simulink model "eAgriBot_V4"  (R2022b)
settings: Solver=ode3  StartTime=0.0  StopTime=t_sim  FixedStep=step_size  RelTol=1e-3
values from neighbouring files (symbols this model uses):
  accel = 0.1*9.81    (= 0.981)    [Run_eAgriBot_V4.m]
  B_tines = 5    [Run_eAgriBot_V4.m]
  brake_bias = 1    [Run_eAgriBot_V4.m]
  c = 6100    [Run_eAgriBot_V4.m]
  decel = 0.15*9.81    (= 1.4715)    [Run_eAgriBot_V4.m]
  decel_begin_dist = total_dist_target    (= 100)    [Run_eAgriBot_V4.m]
  drivetype = 3    [Run_eAgriBot_V4.m]
  effmap = [0.5 0.586 0.723 0.778 0.614 0.604 0.6 0.584 0.709 0.658 0.586 0.688 ... (121 elements, 11x11)]    [EM_effmap_generic.mat]
  end_delay = 4    [Run_eAgriBot_V4.m]
  F_tines = 5    [Run_eAgriBot_V4.m]
  Fb_max = m*g    (= 5101.2)    [Run_eAgriBot_V4.m]
  FT_c_x_rel = l_f    (= 0.645)    [Run_eAgriBot_V4.m]
  FT_c_z_rel = R_u-h_CoG    (= -0.2825)    [Run_eAgriBot_V4.m]
  g = 9.81    [Run_eAgriBot_V4.m]
  gb_eff = 0.98    [Run_eAgriBot_V4.m]
  ground_coh = c*ones(length(ground_points),1)    [Run_eAgriBot_V4.m]
  ground_dens = gamma_s*ones(length(ground_points),1)    [Run_eAgriBot_V4.m]
  ground_height = zeros(length(ground_points),1)    [Run_eAgriBot_V4.m]
  ground_kxy = k_xy*ones(length(ground_points),1)    [Run_eAgriBot_V4.m]
  ground_res = 0.01    [Run_eAgriBot_V4.m]
  Har_back_tip_x_rel = Har_back_top_x_rel+Har_tine_length*cos(Har_angle)    [Run_eAgriBot_V4.m]
  Har_back_tip_z_rel = abs(Hook_z_rel)-h_CoG-Har_tine_depth    [Run_eAgriBot_V4.m]
  Har_back_top_x_rel = -2.0    (= -2)    [Run_eAgriBot_V4.m]
  Har_back_top_z_rel = Har_back_tip_z_rel+Har_tine_length*sin(Har_angle)    [Run_eAgriBot_V4.m]
  Har_front_tip_x_rel = Har_front_top_x_rel+Har_tine_length*cos(Har_angle)    [Run_eAgriBot_V4.m]
  Har_front_tip_z_rel = abs(Hook_z_rel)-h_CoG-Har_tine_depth    [Run_eAgriBot_V4.m]
  Har_front_top_x_rel = -1.2    [Run_eAgriBot_V4.m]
  Har_front_top_z_rel = Har_front_tip_z_rel+Har_tine_length*sin(Har_angle)    [Run_eAgriBot_V4.m]
  Har_tine_length = 0.25    [Run_eAgriBot_V4.m]
  Har_tine_width = 0.02    [Run_eAgriBot_V4.m]
  Har_tire_rad = 0.5842/2    (= 0.2921)    [Run_eAgriBot_V4.m]
  Har_tire_x_rel = -1.5    [Run_eAgriBot_V4.m]
  Har_tire_z_rel = abs(Hook_z_rel)-h_CoG+Har_tire_rad    [Run_eAgriBot_V4.m]
  Hook_x_rel = l_f-l-0.4    (= -1.045)    [Run_eAgriBot_V4.m]
  Hook_z_rel = -0.3    [Run_eAgriBot_V4.m]
  i_front = 17.9542    [Run_eAgriBot_V4.m]
  I_gain = 0.0    (= 0)    [Run_eAgriBot_V4.m]
  i_rear = 17.9542    [Run_eAgriBot_V4.m]
  I_y = 150    [Run_eAgriBot_V4.m]
  I_y_tool = 20    [Run_eAgriBot_V4.m]
  index_init = round(FT_init_exit_x/ground_res)+1    [Run_eAgriBot_V4.m]
  init_CoG_height = h_CoG-0.001    (= 0.599)    [Run_eAgriBot_V4.m]
  init_CoG_v_z = 0    [Run_eAgriBot_V4.m]
  init_omega = 0    [Run_eAgriBot_V4.m]
  init_theta = 0    [Run_eAgriBot_V4.m]
  J_front = J_drive    (= 15)    [Run_eAgriBot_V4.m]
  J_harrow = 1    [Run_eAgriBot_V4.m]
  J_rear = J_drive    (= 15)    [Run_eAgriBot_V4.m]
  k_d = 50e2    (= 5000)    [Run_eAgriBot_V4.m]
  k_d_har = 50e2    (= 5000)    [Run_eAgriBot_V4.m]
  m = 520    [Run_eAgriBot_V4.m]
  m_tool = 200    [Run_eAgriBot_V4.m]
  main_cycle_delay = 5    [Run_eAgriBot_V4.m]
  mu = 0.35    [Run_eAgriBot_V4.m]
  omega_tool_init = 0    [Run_eAgriBot_V4.m]
  P_aux = 200    [Run_eAgriBot_V4.m]
  P_gain = 1.0    (= 1)    [Run_eAgriBot_V4.m]
  pack_Ah = 360    [Battery_data_V5_Kokam_NMC.mat]
  pack_R_charge = [0.00267222222222 0.00267222222222 0.00317777777778 0.00310555555556 0.0026 0.00281666666667 0.00332222222222 0.00353888888889 0.00325 0.00382777777778 0.00382777777778]    [Battery_data_V5_Kokam_NMC.mat]
  pack_R_discharge = [0.00267222222222 0.00267222222222 0.00317777777778 0.00310555555556 0.0026 0.00281666666667 0.00332222222222 0.00353888888889 0.00325 0.00382777777778 0.00382777777778]    [Battery_data_V5_Kokam_NMC.mat]
  pack_VOC = [54.509 52.351 50.895 49.556 48.477 47.645 47.008 46.449 45.825 44.941 44.941]    [Battery_data_V5_Kokam_NMC.mat]
  params2 = [exit_angle reso theta_m_max s_d_tol po]    [Run_eAgriBot_V4.m]
  phi = 26.6    [Run_eAgriBot_V4.m]
  pre_accel = 0.1*9.81    (= 0.981)    [Run_eAgriBot_V4.m]
  pre_decel = 0.15*9.81    (= 1.4715)    [Run_eAgriBot_V4.m]
  pre_decel_begin_dist = pre_dist_target-pre_decel_dist    (= 2.34454218631)    [Run_eAgriBot_V4.m]
  pre_vel = 5    [Run_eAgriBot_V4.m]
  r_front = R_u    (= 0.3175)    [Run_eAgriBot_V4.m]
  r_rear = R_u    (= 0.3175)    [Run_eAgriBot_V4.m]
  rho_t = gamma_s/9.81    (= 1664.01630989)    [Run_eAgriBot_V4.m]
  RT_c_x_rel = l_f-l    (= -0.645)    [Run_eAgriBot_V4.m]
  RT_c_z_rel = R_u-h_CoG    (= -0.2825)    [Run_eAgriBot_V4.m]
  s_init = 3    [Run_eAgriBot_V4.m]
  simu_max_time = cycle_total_time*4    (= 259.930519878)    [Run_eAgriBot_V4.m]
  slip_init = 0    [Run_eAgriBot_V4.m]
  slip_ub = r_rear*1.75    (= 0.555625)    [Run_eAgriBot_V4.m]
  slip_ub_har = Har_tire_rad*1.90    (= 0.55499)    [Run_eAgriBot_V4.m]
  SOC_init = 0.8    [Run_eAgriBot_V4.m]
  SOD = [0 0.1 0.2 0.3 0.4 0.5 0.6 0.7 0.8 0.9 1]    [Battery_data_V5_Kokam_NMC.mat]
  sr_lim_skid = -0.2    [Run_eAgriBot_V4.m]
  sr_lim_slip_f = 0.20-slip_trig    (= 0.18)    [Run_eAgriBot_V4.m]
  sr_lim_slip_r = 0.14-slip_trig    (= 0.12)    [Run_eAgriBot_V4.m]
  step_size = 1e-3    (= 0.001)    [Run_eAgriBot_V4.m]
  T = [80 80 75 70.5882352941 66.6666666667 63.1578947368 60 57.1428571429 54.5454545455 52.1739130435 50 48 ... (49 elements, 49x1)]    [EM_data_V4.mat]    (also in Run_eAgriBot_V4.m = 2*T)
  T_effmap = [0 8 16 24 32 40 48 56 64 72 80]    [EM_effmap_generic.mat]    (also in Run_eAgriBot_V4.m = 2*T_effmap)
  T_multi_r = 1.5    [Run_eAgriBot_V4.m]
  t_params = [c k_c k_phi phi k_xy gamma_s R_u wid c_0 c_1 c_0f c_1f n_0 n_1 k_1 k_2 k_3]    [Run_eAgriBot_V4.m]
  t_params_har = [c k_c k_phi phi k_xy gamma_s Har_tire_rad Har_tire_wid c_0 c_1 c_0f c_1f n_0 n_1 k_1 k_2 k_3]    [Run_eAgriBot_V4.m]
  theta_tool_init = 0    [Run_eAgriBot_V4.m]
  Tine_vz_damping = 0    [Run_eAgriBot_V4.m]
  Tool_x_rel = -1.3    [Run_eAgriBot_V4.m]
  Tool_z_rel = -0.08    [Run_eAgriBot_V4.m]
  v_init = 0    [Run_eAgriBot_V4.m]
  vel_max = 8    [Run_eAgriBot_V4.m]
  w = [0 75 80 85 90 95 100 105 110 115 120 125 ... (49 elements, 49x1)]    [EM_data_V4.mat]
  w_effmap = [0 31.4159265359 62.8318530718 94.2477796077 125.663706144 157.079632679 188.495559215 219.911485751 251.327412287 282.743338823 314.159265359]    [EM_effmap_generic.mat]
libraries: slpidlib x1, simulink x1
(part 1 of 4)
settings Model: Creator=kivek  LastModifiedBy=kivek
settings DataIOCC: ReturnWorkspaceOutputs=off
settings DebuggingCC: UnconnectedInputMsg=warning  UnconnectedOutputMsg=warning  UnconnectedLineMsg=warning
settings ModelReferenceCC: EnableRefExpFcnMdlSchedulingChecks=on
settings RTWCC: DLArmComputeVersion=19.05

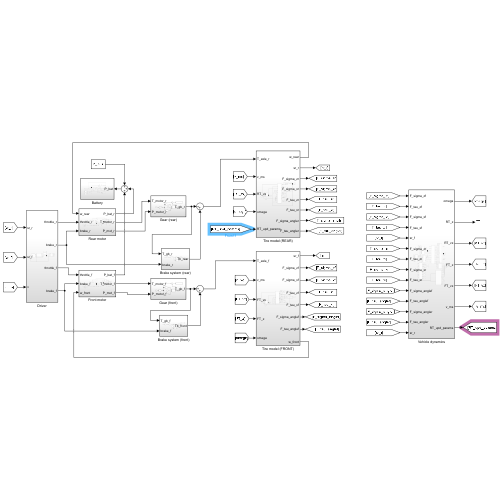
[thumbnail: Simulink's stored preview of the top-level diagram]
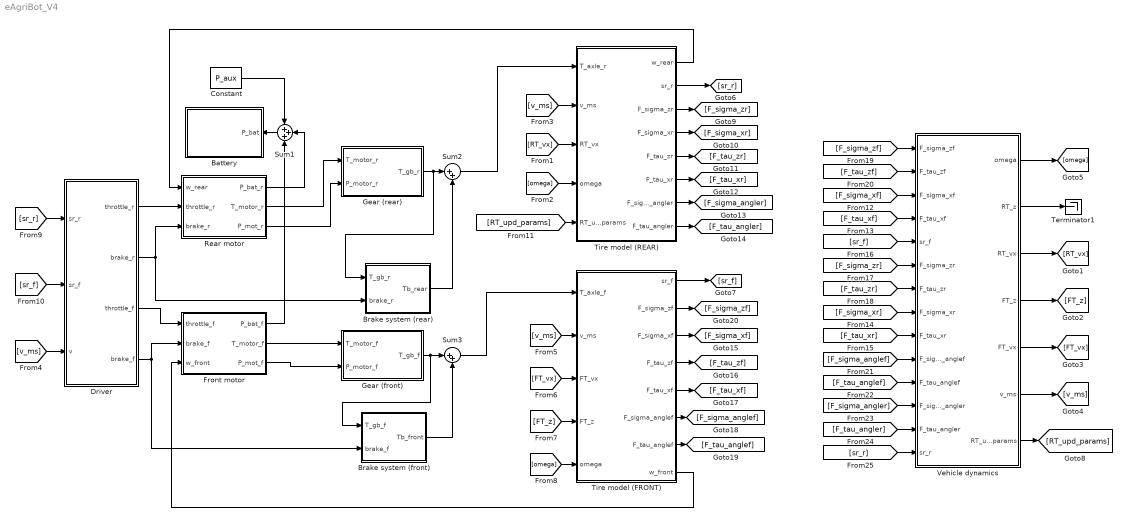
== system eAgriBot_V4 ==
  Battery : Subsystem
  Brake system (front) : Subsystem
  Brake system (rear) : Subsystem
  Constant : Constant  Value=P_aux
  Driver : Subsystem
  Front motor : Subsystem
  Gear (front) : Subsystem
  Gear (rear) : Subsystem
  Rear motor : Subsystem
  Sum1 : Sum  Inputs=+++
  Sum2 : Sum  Inputs=|++
  Sum3 : Sum  Inputs=|++
  Terminator1 : Terminator
  Tire model (FRONT) : Subsystem
  Tire model (REAR) : Subsystem
  Vehicle dynamics : Subsystem
  wires:
  Rear motor/2(T_motor_r) -> Gear (rear)/1(T_motor_r)
  Tire model (REAR)/1(w_rear) -> Rear motor/1(w_rear)
  Driver/1(throttle_r) -> Rear motor/2(throttle_r)
  Driver/2(brake_r) -> Brake system (rear)/2(brake_r), Rear motor/3(brake_r)
  Gear (rear)/1(T_gb_r) -> Brake system (rear)/1(T_gb_r), Sum2/1
  Brake system (rear)/1(Tb_rear) -> Sum2/2
  Sum2/1 -> Tire model (REAR)/1(T_axle_r)
  Vehicle dynamics/2(RT_z) -> Terminator1/1
  [RT_vx] -> Tire model (REAR)/3(RT_vx)
  [omega] -> Tire model (REAR)/4(omega)
  Vehicle dynamics/3(RT_vx) -> [RT_vx]
  Vehicle dynamics/4(FT_z) -> [FT_z]
  Vehicle dynamics/5(FT_vx) -> [FT_vx]
  Vehicle dynamics/6(v_ms) -> [v_ms]
  [v_ms] -> Tire model (REAR)/2(v_ms)
  Vehicle dynamics/1(omega) -> [omega]
  [v_ms] -> Driver/3(v)
  [v_ms] -> Tire model (FRONT)/2(v_ms)
  [FT_vx] -> Tire model (FRONT)/3(FT_vx)
  [FT_z] -> Tire model (FRONT)/4(FT_z)
  [omega] -> Tire model (FRONT)/5(omega)
  Tire model (REAR)/2(sr_r) -> [sr_r]
  [sr_r] -> Driver/1(sr_r)
  Vehicle dynamics/7(RT_upd_params) -> [RT_upd_params]
  [RT_upd_params] -> Tire model (REAR)/5(RT_upd_params)
  Tire model (REAR)/3(F_sigma_zr) -> [F_sigma_zr]
  Tire model (REAR)/4(F_sigma_xr) -> [F_sigma_xr]
  Tire model (REAR)/5(F_tau_zr) -> [F_tau_zr]
  Tire model (REAR)/6(F_tau_xr) -> [F_tau_xr]
  Tire model (REAR)/7(F_sigma_angler) -> [F_sigma_angler]
  Tire model (REAR)/8(F_tau_angler) -> [F_tau_angler]
  Tire model (FRONT)/1(sr_f) -> [sr_f]
  Tire model (FRONT)/4(F_tau_zf) -> [F_tau_zf]
  Tire model (FRONT)/5(F_tau_xf) -> [F_tau_xf]
  Tire model (FRONT)/6(F_sigma_anglef) -> [F_sigma_anglef]
  Tire model (FRONT)/7(F_tau_anglef) -> [F_tau_anglef]
  Tire model (FRONT)/2(F_sigma_zf) -> [F_sigma_zf]
  Tire model (FRONT)/3(F_sigma_xf) -> [F_sigma_xf]
  [F_sigma_xf] -> Vehicle dynamics/3(F_sigma_xf)
  [F_tau_xf] -> Vehicle dynamics/4(F_tau_xf)
  [F_sigma_xr] -> Vehicle dynamics/8(F_sigma_xr)
  [F_tau_xr] -> Vehicle dynamics/9(F_tau_xr)
  [sr_f] -> Vehicle dynamics/5(sr_f)
  [F_sigma_zr] -> Vehicle dynamics/6(F_sigma_zr)
  [F_tau_zr] -> Vehicle dynamics/7(F_tau_zr)
  [F_sigma_zf] -> Vehicle dynamics/1(F_sigma_zf)
  [F_tau_zf] -> Vehicle dynamics/2(F_tau_zf)
  [F_sigma_anglef] -> Vehicle dynamics/10(F_sigma_anglef)
  [F_tau_anglef] -> Vehicle dynamics/11(F_tau_anglef)
  [F_sigma_angler] -> Vehicle dynamics/12(F_sigma_angler)
  [F_tau_angler] -> Vehicle dynamics/13(F_tau_angler)
  [sr_r] -> Vehicle dynamics/14(sr_r)
  [sr_f] -> Driver/2(sr_f)
  Sum1/1 -> Battery/1(P_bat)
  Rear motor/1(P_bat_r) -> Sum1/2
  Tire model (FRONT)/8(w_front) -> Front motor/3(w_front)
  Driver/3(throttle_f) -> Front motor/1(throttle_f)
  Driver/4(brake_f) -> Brake system (front)/2(brake_f), Front motor/2(brake_f)
  Front motor/2(T_motor_f) -> Gear (front)/1(T_motor_f)
  Gear (front)/1(T_gb_f) -> Brake system (front)/1(T_gb_f), Sum3/1
  Sum3/1 -> Tire model (FRONT)/1(T_axle_f)
  Brake system (front)/1(Tb_front) -> Sum3/2
  Rear motor/3(P_mot_r) -> Gear (rear)/2(P_motor_r)
  Front motor/3(P_mot_f) -> Gear (front)/2(P_motor_f)
  Front motor/1(P_bat_f) -> Sum1/3
  Constant/1 -> Sum1/1

== system eAgriBot_V4/Battery ==
  P_bat : Inport
  Constant : Constant  Value=pack_Ah
  Constant1 : Constant
  Divide : Product  Inputs=*/
  Divide1 : Product  Inputs=*/
  Gain : Gain  Gain=4
  Gain1 : Gain  Gain=2
  Gain2 : Gain  Gain=3600
  Gain3 : Gain  Gain=100
  Integrator : Integrator  InitialCondition=1-SOC_init
  Integrator1 : Integrator
  Integrator2 : Integrator
  Product : Product
  Product1 : Product
  Product2 : Product
  R_charge : Lookup_n-D  NumberOfTableDimensions=1  BreakpointsForDimension1=SOD  Table=pack_R_charge  InternalRulePriority=Speed  RndMeth=Simplest
  R_discharge : Lookup_n-D  NumberOfTableDimensions=1  BreakpointsForDimension1=SOD  Table=pack_R_discharge  InternalRulePriority=Speed  RndMeth=Simplest
  Scope2 : Scope
  Sqrt : Sqrt
  Square : Math  Operator=square
  Square1 : Math  Operator=square
  Sum : Sum  Inputs=|+-
  Sum1 : Sum  Inputs=+-|
  Sum2 : Sum  Inputs=-+|
  Switch : Switch  SaturateOnIntegerOverflow=off  InputSameDT=off
  To Workspace : ToWorkspace  VariableName=Bat_energy_consumption  SaveFormat=Timeseries  SampleTime=-1
  To Workspace1 : ToWorkspace  VariableName=Bat_internal_losses  SaveFormat=Timeseries  SampleTime=-1
  To Workspace2 : ToWorkspace  VariableName=Bat_soc  SaveFormat=Timeseries  SampleTime=-1
  To Workspace3 : ToWorkspace  VariableName=Bat_loss_power  SaveFormat=Timeseries  SampleTime=-1
  U_voc : Lookup_n-D  NumberOfTableDimensions=1  BreakpointsForDimension1=SOD  Table=pack_VOC  InternalRulePriority=Speed  RndMeth=Simplest
  wires:
  Constant1/1 -> Sum2/2
  Constant/1 -> Gain2/1
  P_bat/1 -> Switch/2, Product/1
  U_voc/1 -> Product1/1, Sum1/1, Square/1
  Gain1/1 -> Divide/2
  Integrator/1 -> Sum2/1, R_charge/1, R_discharge/1, U_voc/1
  Square/1 -> Sum/1
  Sum2/1 -> Gain3/1
  Product/1 -> Gain/1
  Sum/1 -> Sqrt/1
  Gain/1 -> Sum/2
  Divide/1 -> Square1/1, Product1/2, Divide1/1
  Product1/1 -> Integrator1/1
  Divide1/1 -> Integrator/1
  Integrator1/1 -> To Workspace/1
  Sum1/1 -> Divide/1
  Gain2/1 -> Divide1/2
  Gain3/1 -> To Workspace2/1
  Sqrt/1 -> Sum1/2
  Square1/1 -> Product2/1
  Product2/1 -> To Workspace3/1, Integrator2/1
  Integrator2/1 -> To Workspace1/1
  Switch/1 -> Scope2/1, Gain1/1, Product2/2, Product/2
  R_discharge/1 -> Switch/1
  R_charge/1 -> Switch/3

== system eAgriBot_V4/Brake system (front) ==
  T_gb_f : Inport
  brake_f : Inport  Port=2
  Constant : Constant  Value=0
  Gain1 : Gain  Gain=Fb_max
  Gain2 : Gain  Gain=r_front
  Gain4 : Gain  Gain=brake_bias
  Saturation1 : Saturate  UpperLimit=0  LowerLimit=-inf
  Sum : Sum  Inputs=|+-
  Switch : Switch  SaturateOnIntegerOverflow=off  InputSameDT=off
  To Workspace : ToWorkspace  VariableName=brake_torque_front  SaveFormat=Timeseries  SampleTime=-1
  Tb_front : Outport
  wires:
  brake_f/1 -> Gain1/1
  Gain4/1 -> Gain2/1
  Gain1/1 -> Gain4/1
  Saturation1/1 -> Tb_front/1, To Workspace/1
  Constant/1 -> Switch/1
  Switch/1 -> Sum/2
  T_gb_f/1 -> Switch/3, Switch/2
  Gain2/1 -> Sum/1
  Sum/1 -> Saturation1/1

== system eAgriBot_V4/Brake system (rear) ==
  T_gb_r : Inport
  brake_r : Inport  Port=2
  Constant : Constant  Value=0
  Gain1 : Gain  Gain=Fb_max
  Gain3 : Gain  Gain=r_rear
  Gain5 : Gain  Gain=1-brake_bias
  Saturation : Saturate  UpperLimit=0  LowerLimit=-inf
  Sum : Sum  Inputs=|+-
  Switch : Switch  SaturateOnIntegerOverflow=off  InputSameDT=off
  To Workspace2 : ToWorkspace  VariableName=brake_torque_rear  SaveFormat=Timeseries  SampleTime=-1
  Tb_rear : Outport
  wires:
  Gain5/1 -> Gain3/1
  brake_r/1 -> Gain1/1
  Gain1/1 -> Gain5/1
  T_gb_r/1 -> Switch/3, Switch/2
  Constant/1 -> Switch/1
  Gain3/1 -> Sum/1
  Switch/1 -> Sum/2
  Sum/1 -> Saturation/1
  Saturation/1 -> Tb_rear/1, To Workspace2/1

== system eAgriBot_V4/Driver ==
  sr_r : Inport
  sr_f : Inport  Port=2
  v : Inport  Port=3
  Control : Subsystem
  Cycle selection : Switch  SaturateOnIntegerOverflow=off  InputSameDT=off
  Main cycle : Subsystem
  Pre-cycle : Subsystem
  Stop simulation : Subsystem
  Sum : Sum  Inputs=|+-
  To Workspace3 : ToWorkspace  VariableName=v_ms_cycle  SaveFormat=Timeseries  SampleTime=-1
  throttle_r : Outport
  brake_r : Outport  Port=2
  throttle_f : Outport  Port=3
  brake_f : Outport  Port=4
  wires:
  v/1 -> Pre-cycle/1(v_ms), Main cycle/2(v_ms), Sum/2
  Cycle selection/1 -> Sum/1, To Workspace3/1, Control/3(v_ref)
  Pre-cycle/2(v_ref_precycle) -> Cycle selection/3
  Pre-cycle/1(end_time_new) -> Main cycle/1(end_time_precycle)
  Main cycle/2(v_ref_maincycle) -> Cycle selection/1
  Main cycle/3(main_cycle_on_check) -> Cycle selection/2
  Main cycle/1(end_time_new) -> Stop simulation/1(main_cycle_endtime)
  sr_r/1 -> Control/1(sr_r)
  Sum/1 -> Control/4(v_error)
  Control/1(throttle_r) -> throttle_r/1
  Control/2(brake_r) -> brake_r/1
  sr_f/1 -> Control/2(sr_f)
  Control/3(throttle_f) -> throttle_f/1
  Control/4(brake_f) -> brake_f/1

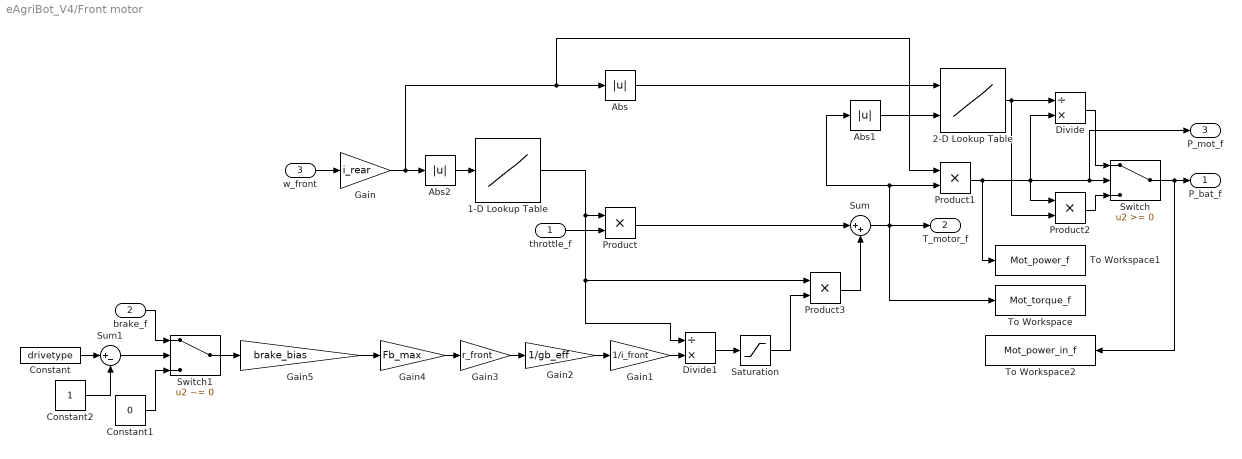
== system eAgriBot_V4/Front motor ==
  throttle_f : Inport
  brake_f : Inport  Port=2
  w_front : Inport  Port=3
  1-D Lookup Table : Lookup_n-D  NumberOfTableDimensions=1  BreakpointsForDimension1=w  Table=T  InternalRulePriority=Speed  RndMeth=Simplest
  2-D Lookup Table : Lookup_n-D  BreakpointsForDimension1=w_effmap  BreakpointsForDimension2=T_effmap  Table=effmap  InternalRulePriority=Speed  RndMeth=Simplest
      settings: InputPortMap=u0,u1
  Abs : Abs  SaturateOnIntegerOverflow=off
  Abs1 : Abs  SaturateOnIntegerOverflow=off
  Abs2 : Abs  SaturateOnIntegerOverflow=off
  Constant : Constant  Value=drivetype
  Constant1 : Constant  Value=0
  Constant2 : Constant
  Divide : Product  Inputs=/*
  Divide1 : Product  Inputs=/*
  Gain : Gain  Gain=i_rear
  Gain1 : Gain  Gain=1/i_front
  Gain2 : Gain  Gain=1/gb_eff
  Gain3 : Gain  Gain=r_front
  Gain4 : Gain  Gain=Fb_max
  Gain5 : Gain  Gain=brake_bias
  Product{,1..3} (4 alike) : Product
  Saturation : Saturate  UpperLimit=0  LowerLimit=-1
  Sum : Sum  Inputs=|++
  Sum1 : Sum  Inputs=|+-
  Switch : Switch  SaturateOnIntegerOverflow=off  InputSameDT=off
  Switch1 : Switch  Criteria=u2 ~= 0  SaturateOnIntegerOverflow=off  InputSameDT=off
  To Workspace : ToWorkspace  VariableName=Mot_torque_f  SaveFormat=Timeseries  SampleTime=-1
  To Workspace1 : ToWorkspace  VariableName=Mot_power_f  SaveFormat=Timeseries  SampleTime=-1
  To Workspace2 : ToWorkspace  VariableName=Mot_power_in_f  SaveFormat=Timeseries  SampleTime=-1
  P_bat_f : Outport
  T_motor_f : Outport  Port=2
  P_mot_f : Outport  Port=3
  wires:
  throttle_f/1 -> Product/2
  w_front/1 -> Gain/1
  1-D Lookup Table/1 -> Product/1, Product3/1, Divide1/1
  Gain/1 -> Abs2/1, Abs/1, Product1/1
  Product1/1 -> To Workspace1/1, Product2/1, Divide/2, P_mot_f/1, Switch/2
  2-D Lookup Table/1 -> Product2/2, Divide/1
  Divide/1 -> Switch/1
  Product2/1 -> Switch/3
  Switch/1 -> To Workspace2/1, P_bat_f/1
  Sum/1 -> To Workspace/1, Abs1/1, Product1/2, T_motor_f/1
  Product/1 -> Sum/1
  Product3/1 -> Sum/2
  Abs/1 -> 2-D Lookup Table/1
  Abs1/1 -> 2-D Lookup Table/2
  Gain4/1 -> Gain3/1
  Gain3/1 -> Gain2/1
  Gain2/1 -> Gain1/1
  Gain1/1 -> Divide1/2
  Divide1/1 -> Saturation/1
  Saturation/1 -> Product3/2
  Gain5/1 -> Gain4/1
  Constant2/1 -> Sum1/2
  Sum1/1 -> Switch1/2
  Constant1/1 -> Switch1/3
  Constant/1 -> Sum1/1
  brake_f/1 -> Switch1/1
  Switch1/1 -> Gain5/1
  Abs2/1 -> 1-D Lookup Table/1

== system eAgriBot_V4/Gear (front) ==
  T_motor_f : Inport
  P_motor_f : Inport  Port=2
  Gain : Gain  Gain=i_front
  Gain1 : Gain  Gain=gb_eff
  Gain2 : Gain  Gain=1/gb_eff
  Sum : Sum  Inputs=|+-
  Switch : Switch  SaturateOnIntegerOverflow=off  InputSameDT=off
  To Workspace : ToWorkspace  VariableName=T_loss_gb_f  SaveFormat=Timeseries  SampleTime=-1
  T_gb_f : Outport
  wires:
  T_motor_f/1 -> Gain/1
  Switch/1 -> Sum/2, T_gb_f/1
  P_motor_f/1 -> Switch/2
  Gain1/1 -> Switch/1
  Gain/1 -> Gain2/1, Sum/1, Gain1/1
  Gain2/1 -> Switch/3
  Sum/1 -> To Workspace/1

== system eAgriBot_V4/Gear (rear) ==
  T_motor_r : Inport
  P_motor_r : Inport  Port=2
  Gain : Gain  Gain=i_rear
  Gain1 : Gain  Gain=gb_eff
  Gain3 : Gain  Gain=1/gb_eff
  Sum : Sum  Inputs=|+-
  Switch : Switch  SaturateOnIntegerOverflow=off  InputSameDT=off
  To Workspace : ToWorkspace  VariableName=T_loss_gb_r  SaveFormat=Timeseries  SampleTime=-1
  T_gb_r : Outport
  wires:
  T_motor_r/1 -> Gain/1
  P_motor_r/1 -> Switch/2
  Switch/1 -> Sum/2, T_gb_r/1
  Gain1/1 -> Switch/1
  Gain/1 -> Gain3/1, Sum/1, Gain1/1
  Gain3/1 -> Switch/3
  Sum/1 -> To Workspace/1

== system eAgriBot_V4/Rear motor ==
  w_rear : Inport
  throttle_r : Inport  Port=2
  brake_r : Inport  Port=3
  1-D Lookup Table : Lookup_n-D  NumberOfTableDimensions=1  BreakpointsForDimension1=w  Table=T  InternalRulePriority=Speed  RndMeth=Simplest
  2-D Lookup Table : Lookup_n-D  BreakpointsForDimension1=w_effmap  BreakpointsForDimension2=T_effmap  Table=effmap  InternalRulePriority=Speed  RndMeth=Simplest
      settings: InputPortMap=u0,u1
  Abs : Abs  SaturateOnIntegerOverflow=off
  Abs1 : Abs  SaturateOnIntegerOverflow=off
  Abs2 : Abs  SaturateOnIntegerOverflow=off
  Constant : Constant  Value=drivetype
  Constant1 : Constant  Value=0
  Constant2 : Constant  Value=2
  Divide : Product  Inputs=/*
  Divide1 : Product  Inputs=/*
  Gain : Gain  Gain=i_rear
  Gain1 : Gain  Gain=1/i_rear
  Gain2 : Gain  Gain=1/gb_eff
  Gain3 : Gain  Gain=r_rear
  Gain4 : Gain  Gain=Fb_max
  Gain5 : Gain  Gain=1-brake_bias
  Product{,1..3} (4 alike) : Product
  Saturation : Saturate  UpperLimit=0  LowerLimit=-1
  Sum : Sum  Inputs=|++
  Sum1 : Sum  Inputs=|+-
  Switch : Switch  SaturateOnIntegerOverflow=off  InputSameDT=off
  Switch1 : Switch  Criteria=u2 ~= 0  SaturateOnIntegerOverflow=off  InputSameDT=off
  To Workspace : ToWorkspace  VariableName=Mot_torque  SaveFormat=Timeseries  SampleTime=-1
  To Workspace1 : ToWorkspace  VariableName=Mot_power  SaveFormat=Timeseries  SampleTime=-1
  To Workspace2 : ToWorkspace  VariableName=Mot_power_in_r  SaveFormat=Timeseries  SampleTime=-1
  P_bat_r : Outport
  T_motor_r : Outport  Port=2
  P_mot_r : Outport  Port=3
  wires:
  throttle_r/1 -> Product/2
  w_rear/1 -> Gain/1
  1-D Lookup Table/1 -> Product/1, Product3/1, Divide1/1
  Gain/1 -> Abs2/1, Product1/1, Abs/1
  Product1/1 -> To Workspace1/1, Product2/1, Divide/2, P_mot_r/1, Switch/2
  2-D Lookup Table/1 -> Product2/2, Divide/1
  Divide/1 -> Switch/1
  Product2/1 -> Switch/3
  Switch/1 -> To Workspace2/1, P_bat_r/1
  Sum/1 -> To Workspace/1, Abs1/1, Product1/2, T_motor_r/1
  Product/1 -> Sum/1
  Product3/1 -> Sum/2
  Abs/1 -> 2-D Lookup Table/1
  Abs1/1 -> 2-D Lookup Table/2
  Gain4/1 -> Gain3/1
  Gain3/1 -> Gain2/1
  Gain2/1 -> Gain1/1
  Gain1/1 -> Divide1/2
  Divide1/1 -> Saturation/1
  Saturation/1 -> Product3/2
  Gain5/1 -> Gain4/1
  brake_r/1 -> Switch1/1
  Switch1/1 -> Gain5/1
  Constant1/1 -> Switch1/3
  Constant/1 -> Sum1/1
  Constant2/1 -> Sum1/2
  Sum1/1 -> Switch1/2
  Abs2/1 -> 1-D Lookup Table/1

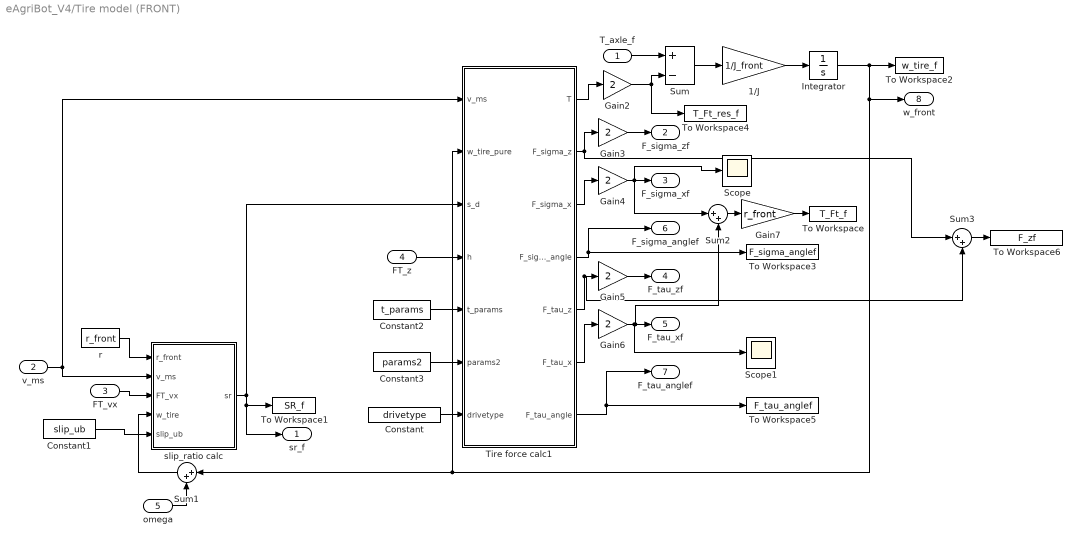
== system eAgriBot_V4/Tire model (FRONT) ==
  T_axle_f : Inport
  v_ms : Inport  Port=2
  FT_vx : Inport  Port=3
  FT_z : Inport  Port=4
  omega : Inport  Port=5
  1/J : Gain  Gain=1/J_front
  Constant : Constant  Value=drivetype
  Constant1 : Constant  Value=slip_ub
  Constant2 : Constant  Value=t_params
  Constant3 : Constant  Value=params2
  Gain{2..6} (5 alike) : Gain  Gain=2
  Gain7 : Gain  Gain=r_front
  Integrator : Integrator  InitialCondition=v_init/r_rear*(1+slip_init)  LimitOutput=on  LowerSaturationLimit=0
  Scope : Scope
  Scope1 : Scope
  Sum : Sum  Inputs=+-
  Sum1 : Sum  Inputs=|++
  Sum2 : Sum  Inputs=|++
  Sum3 : Sum  Inputs=|++
  Tire force calc1 : MATLAB Function  TreatAsAtomicUnit=on  SystemSampleTime=step_size
  To Workspace : ToWorkspace  VariableName=T_Ft_f  SaveFormat=Timeseries  SampleTime=-1
  To Workspace1 : ToWorkspace  VariableName=SR_f  SaveFormat=Timeseries  SampleTime=-1
  To Workspace2 : ToWorkspace  VariableName=w_tire_f  SaveFormat=Timeseries  SampleTime=-1
  To Workspace3 : ToWorkspace  VariableName=F_sigma_anglef  SaveFormat=Timeseries  SampleTime=-1
  To Workspace4 : ToWorkspace  VariableName=T_Ft_res_f  SaveFormat=Timeseries  SampleTime=-1
  To Workspace5 : ToWorkspace  VariableName=F_tau_anglef  SaveFormat=Timeseries  SampleTime=-1
  To Workspace6 : ToWorkspace  VariableName=F_zf  SaveFormat=Timeseries  SampleTime=-1
  r : Constant  Value=r_front
  slip_ratio calc : MATLAB Function  TreatAsAtomicUnit=on  SystemSampleTime=step_size
  sr_f : Outport
  F_sigma_zf : Outport  Port=2
  F_sigma_xf : Outport  Port=3
  F_tau_zf : Outport  Port=4
  F_tau_xf : Outport  Port=5
  F_sigma_anglef : Outport  Port=6
  F_tau_anglef : Outport  Port=7
  w_front : Outport  Port=8
  wires:
  1/J/1 -> Integrator/1
  Sum/1 -> 1/J/1
  T_axle_f/1 -> Sum/1
  v_ms/1 -> Tire force calc1/1(v_ms), slip_ratio calc/2(v_ms)
  slip_ratio calc/1(sr) -> Tire force calc1/3(s_d), sr_f/1, To Workspace1/1
  Tire force calc1/2(F_sigma_z) -> Gain3/1, Sum3/1
  Tire force calc1/1(T) -> Gain2/1
  FT_vx/1 -> slip_ratio calc/3(FT_vx)
  r/1 -> slip_ratio calc/1(r_front)
  Tire force calc1/3(F_sigma_x) -> Gain4/1
  Sum1/1 -> slip_ratio calc/4(w_tire)
  FT_z/1 -> Tire force calc1/4(h)
  Constant2/1 -> Tire force calc1/5(t_params)
  Constant3/1 -> Tire force calc1/6(params2)
  Gain2/1 -> To Workspace4/1, Sum/2
  Gain3/1 -> F_sigma_zf/1
  Tire force calc1/4(F_sigma_angle) -> F_sigma_anglef/1, To Workspace3/1
  Tire force calc1/5(F_tau_z) -> Sum3/2, Gain5/1
  Gain5/1 -> F_tau_zf/1
  Gain6/1 -> Scope1/1, Sum2/2, F_tau_xf/1
  Tire force calc1/6(F_tau_x) -> Gain6/1
  Tire force calc1/7(F_tau_angle) -> F_tau_anglef/1, To Workspace5/1
  Gain4/1 -> Scope/1, Sum2/1, F_sigma_xf/1
  Sum2/1 -> Gain7/1
  Gain7/1 -> To Workspace/1
  Sum3/1 -> To Workspace6/1
  Constant1/1 -> slip_ratio calc/5(slip_ub)
  Integrator/1 -> To Workspace2/1, Sum1/1, Tire force calc1/2(w_tire_pure), w_front/1
  omega/1 -> Sum1/2
  Constant/1 -> Tire force calc1/7(drivetype)

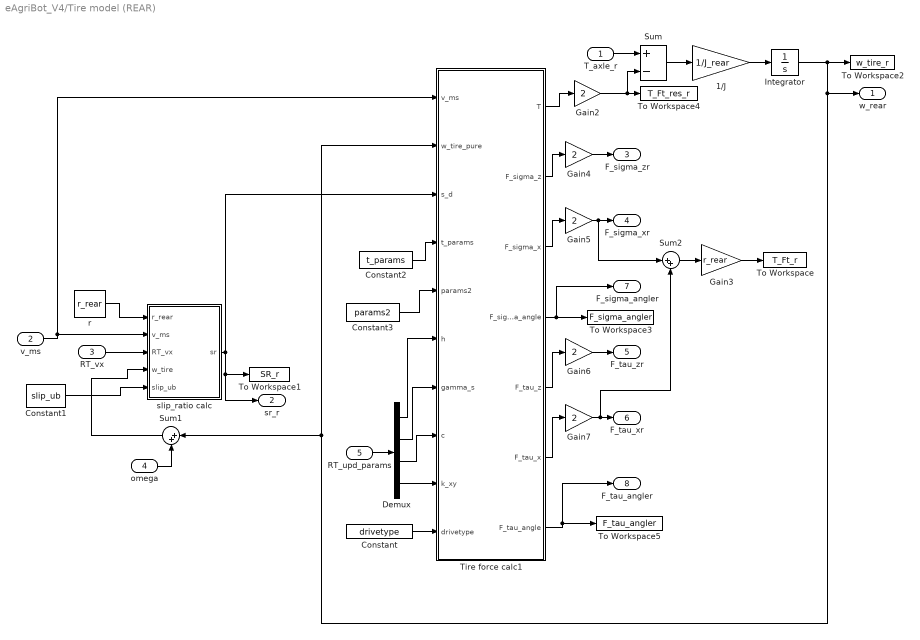
== system eAgriBot_V4/Tire model (REAR) ==
  T_axle_r : Inport
  v_ms : Inport  Port=2
  RT_vx : Inport  Port=3
  omega : Inport  Port=4
  RT_upd_params : Inport  Port=5
  1/J : Gain  Gain=1/J_rear
  Constant : Constant  Value=drivetype
  Constant1 : Constant  Value=slip_ub
  Constant2 : Constant  Value=t_params
  Constant3 : Constant  Value=params2
  Demux : Demux
  Gain{2,4..7} (5 alike) : Gain  Gain=2
  Gain3 : Gain  Gain=r_rear
  Integrator : Integrator  InitialCondition=v_init/r_rear*(1+slip_init)  LimitOutput=on  LowerSaturationLimit=0
  Sum : Sum  Inputs=+-
  Sum1 : Sum  Inputs=|++
  Sum2 : Sum  Inputs=|++
  Tire force calc1 : MATLAB Function  TreatAsAtomicUnit=on  SystemSampleTime=step_size
  To Workspace : ToWorkspace  VariableName=T_Ft_r  SaveFormat=Timeseries  SampleTime=-1
  To Workspace1 : ToWorkspace  VariableName=SR_r  SaveFormat=Timeseries  SampleTime=-1
  To Workspace2 : ToWorkspace  VariableName=w_tire_r  SaveFormat=Timeseries  SampleTime=-1
  To Workspace3 : ToWorkspace  VariableName=F_sigma_angler  SaveFormat=Timeseries  SampleTime=-1
  To Workspace4 : ToWorkspace  VariableName=T_Ft_res_r  SaveFormat=Timeseries  SampleTime=-1
  To Workspace5 : ToWorkspace  VariableName=F_tau_angler  SaveFormat=Timeseries  SampleTime=-1
  r : Constant  Value=r_rear
  slip_ratio calc : MATLAB Function  TreatAsAtomicUnit=on  SystemSampleTime=step_size
  w_rear : Outport
  sr_r : Outport  Port=2
  F_sigma_zr : Outport  Port=3
  F_sigma_xr : Outport  Port=4
  F_tau_zr : Outport  Port=5
  F_tau_xr : Outport  Port=6
  F_sigma_angler : Outport  Port=7
  F_tau_angler : Outport  Port=8
  wires:
  1/J/1 -> Integrator/1
  Sum/1 -> 1/J/1
  T_axle_r/1 -> Sum/1
  v_ms/1 -> Tire force calc1/1(v_ms), slip_ratio calc/2(v_ms)
  Integrator/1 -> To Workspace2/1, Tire force calc1/2(w_tire_pure), Sum1/1, w_rear/1
  Tire force calc1/1(T) -> Gain2/1
  RT_vx/1 -> slip_ratio calc/3(RT_vx)
  r/1 -> slip_ratio calc/1(r_rear)
  omega/1 -> Sum1/2
  Sum1/1 -> slip_ratio calc/4(w_tire)
  Constant2/1 -> Tire force calc1/4(t_params)
  Constant3/1 -> Tire force calc1/5(params2)
  Gain2/1 -> To Workspace4/1, Sum/2
  Gain4/1 -> F_sigma_zr/1
  RT_upd_params/1 -> Demux/1
  Demux/1 -> Tire force calc1/6(h)
  Demux/2 -> Tire force calc1/7(gamma_s)
  Demux/3 -> Tire force calc1/8(c)
  Demux/4 -> Tire force calc1/9(k_xy)
  Tire force calc1/2(F_sigma_z) -> Gain4/1
  Gain5/1 -> Sum2/1, F_sigma_xr/1
  Tire force calc1/3(F_sigma_x) -> Gain5/1
  Gain6/1 -> F_tau_zr/1
  Tire force calc1/5(F_tau_z) -> Gain6/1
  Gain7/1 -> Sum2/2, F_tau_xr/1
  Tire force calc1/6(F_tau_x) -> Gain7/1
  Tire force calc1/4(F_sigma_angle) -> F_sigma_angler/1, To Workspace3/1
  Tire force calc1/7(F_tau_angle) -> F_tau_angler/1, To Workspace5/1
  Sum2/1 -> Gain3/1
  Gain3/1 -> To Workspace/1
  Constant1/1 -> slip_ratio calc/5(slip_ub)
  slip_ratio calc/1(sr) -> sr_r/1, To Workspace1/1, Tire force calc1/3(s_d)
  Constant/1 -> Tire force calc1/10(drivetype)

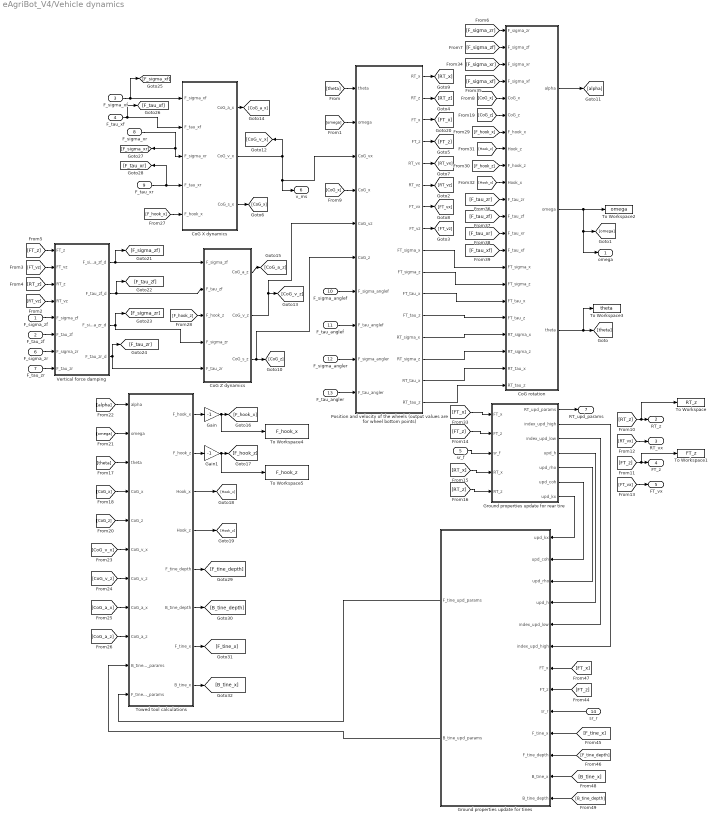
== system eAgriBot_V4/Vehicle dynamics ==
  F_sigma_zf : Inport
  F_tau_zf : Inport  Port=2
  F_sigma_xf : Inport  Port=3
  F_tau_xf : Inport  Port=4
  sr_f : Inport  Port=5
  F_sigma_zr : Inport  Port=6
  F_tau_zr : Inport  Port=7
  F_sigma_xr : Inport  Port=8
  F_tau_xr : Inport  Port=9
  F_sigma_anglef : Inport  Port=10
  F_tau_anglef : Inport  Port=11
  F_sigma_angler : Inport  Port=12
  F_tau_angler : Inport  Port=13
  sr_r : Inport  Port=14
  CoG X dynamics : Subsystem
  CoG Z dynamics : Subsystem
  CoG rotation : Subsystem
  Gain : Gain  Gain=-1
  Gain1 : Gain  Gain=-1
  Ground properties update for rear tire : Subsystem
  Ground properties update for tines : Subsystem
  Position and velocity of the wheels (output values are for wheel bottom points) : Subsystem
  To Workspace : ToWorkspace  VariableName=RT_z  SaveFormat=Timeseries  SampleTime=-1
  To Workspace1 : ToWorkspace  VariableName=FT_z  SaveFormat=Timeseries  SampleTime=-1
  To Workspace2 : ToWorkspace  VariableName=omega  SaveFormat=Timeseries  SampleTime=-1
  To Workspace3 : ToWorkspace  VariableName=theta  SaveFormat=Timeseries  SampleTime=-1
  To Workspace4 : ToWorkspace  VariableName=F_hook_x  SaveFormat=Timeseries  SampleTime=-1
  To Workspace5 : ToWorkspace  VariableName=F_hook_z  SaveFormat=Timeseries  SampleTime=-1
  Towed tool calculations : Subsystem
  Vertical force damping : Subsystem
  omega : Outport
  RT_z : Outport  Port=2
  RT_vx : Outport  Port=3
  FT_z : Outport  Port=4
  FT_vx : Outport  Port=5
  v_ms : Outport  Port=6
  RT_upd_params : Outport  Port=7
  wires:
  F_sigma_xf/1 -> [F_sigma_xf], CoG X dynamics/1(F_sigma_xf)
  F_tau_xf/1 -> [F_tau_xf], CoG X dynamics/2(F_tau_xf)
  CoG X dynamics/2(CoG_v_x) -> [CoG_v_x], v_ms/1, Position and velocity of the wheels (output values are for wheel bottom points)/3(CoG_vx)
  CoG Z dynamics/2(CoG_v_z) -> [CoG_v_z], Position and velocity of the wheels (output values are for wheel bottom points)/5(CoG_vz)
  CoG Z dynamics/3(CoG_s_z) -> Position and velocity of the wheels (output values are for wheel bottom points)/6(CoG_z), [CoG_z]
  Position and velocity of the wheels (output values are for wheel bottom points)/1(RT_x) -> [RT_x]
  CoG rotation/3(theta) -> To Workspace3/1, [theta]
  [theta] -> Position and velocity of the wheels (output values are for wheel bottom points)/1(theta)
  CoG rotation/2(omega) -> omega/1, [omega], To Workspace2/1
  [omega] -> Position and velocity of the wheels (output values are for wheel bottom points)/2(omega)
  Position and velocity of the wheels (output values are for wheel bottom points)/6(RT_vz) -> [RT_vz]
  Position and velocity of the wheels (output values are for wheel bottom points)/8(FT_vz) -> [FT_vz]
  [FT_vz] -> Vertical force damping/2(FT_vz)
  Position and velocity of the wheels (output values are for wheel bottom points)/2(RT_z) -> [RT_z]
  Position and velocity of the wheels (output values are for wheel bottom points)/4(FT_z) -> [FT_z]
  [RT_z] -> Vertical force damping/3(RT_z)
  [FT_z] -> Vertical force damping/1(FT_z)
  [CoG_x] -> CoG rotation/5(CoG_x)
  CoG X dynamics/3(CoG_s_x) -> [CoG_x]
  [CoG_x] -> Position and velocity of the wheels (output values are for wheel bottom points)/4(CoG_x)
  CoG rotation/1(alpha) -> [alpha]
  CoG X dynamics/1(CoG_a_x) -> [CoG_a_x]
  [RT_z] -> To Workspace/1, RT_z/1
  [FT_z] -> To Workspace1/1, FT_z/1
  [RT_vx] -> RT_vx/1
  [FT_vx] -> FT_vx/1
  Position and velocity of the wheels (output values are for wheel bottom points)/5(RT_vx) -> [RT_vx]
  Position and velocity of the wheels (output values are for wheel bottom points)/7(FT_vx) -> [FT_vx]
  [FT_z] -> Ground properties update for rear tire/2(FT_z)
  sr_f/1 -> Ground properties update for rear tire/3(sr_f)
  [RT_x] -> Ground properties update for rear tire/4(RT_x)
  [RT_z] -> Ground properties update for rear tire/5(RT_z)
  Ground properties update for rear tire/1(RT_upd_params) -> RT_upd_params/1
  [theta] -> Towed tool calculations/3(theta)
  [CoG_x] -> Towed tool calculations/4(CoG_x)
  [CoG_z] -> CoG rotation/6(CoG_z)
  [CoG_z] -> Towed tool calculations/5(CoG_z)
  [omega] -> Towed tool calculations/2(omega)
  [alpha] -> Towed tool calculations/1(alpha)
  [CoG_v_x] -> Towed tool calculations/6(CoG_v_x)
  [CoG_v_z] -> Towed tool calculations/7(CoG_v_z)
  [CoG_a_x] -> Towed tool calculations/8(CoG_a_x)
  [CoG_a_z] -> Towed tool calculations/9(CoG_a_z)
  CoG Z dynamics/1(CoG_a_z) -> [CoG_a_z]
  Gain/1 -> To Workspace4/1, [F_hook_x]
  [F_hook_x] -> CoG X dynamics/5(F_hook_x)
  Gain1/1 -> To Workspace5/1, [F_hook_z]
  [F_hook_z] -> CoG Z dynamics/3(F_hook_z)
  [F_hook_x] -> CoG rotation/7(F_hook_x)
  [F_hook_z] -> CoG rotation/9(F_hook_z)
  [Hook_z] -> CoG rotation/8(Hook_z)
  [Hook_x] -> CoG rotation/10(Hook_x)
  Towed tool calculations/3(Hook_x) -> [Hook_x]
  Towed tool calculations/4(Hook_z) -> [Hook_z]
  F_sigma_xr/1 -> CoG X dynamics/3(F_sigma_xr), [F_sigma_xr]
  F_tau_xr/1 -> CoG X dynamics/4(F_tau_xr), [F_tau_xr]
  [RT_vz] -> Vertical force damping/4(RT_vz)
  F_sigma_zf/1 -> Vertical force damping/5(F_sigma_zf)
  F_tau_zf/1 -> Vertical force damping/6(F_tau_zf)
  F_sigma_zr/1 -> Vertical force damping/7(F_sigma_zr)
  F_tau_zr/1 -> Vertical force damping/8(F_tau_zr)
  Vertical force damping/1(F_sigma_zf_d) -> [F_sigma_zf], CoG Z dynamics/1(F_sigma_zf)
  Vertical force damping/2(F_tau_zf_d) -> [F_tau_zf], CoG Z dynamics/2(F_tau_zf)
  Vertical force damping/3(F_sigma_zr_d) -> [F_sigma_zr], CoG Z dynamics/4(F_sigma_zr)
  Vertical force damping/4(F_tau_zr_d) -> [F_tau_zr], CoG Z dynamics/5(F_tau_zr)
  Position and velocity of the wheels (output values are for wheel bottom points)/3(FT_x) -> [FT_x]
  [FT_x] -> Ground properties update for rear tire/1(FT_x)
  Position and velocity of the wheels (output values are for wheel bottom points)/9(FT_sigma_x) -> CoG rotation/15(FT_sigma_x)
  Position and velocity of the wheels (output values are for wheel bottom points)/10(FT_sigma_z) -> CoG rotation/16(FT_sigma_z)
  Position and velocity of the wheels (output values are for wheel bottom points)/11(FT_tau_x) -> CoG rotation/17(FT_tau_x)
  Position and velocity of the wheels (output values are for wheel bottom points)/12(FT_tau_z) -> CoG rotation/18(FT_tau_z)
  Position and velocity of the wheels (output values are for wheel bottom points)/13(RT_sigma_x) -> CoG rotation/19(RT_sigma_x)
  Position and velocity of the wheels (output values are for wheel bottom points)/14(RT_sigma_z) -> CoG rotation/20(RT_sigma_z)
  Position and velocity of the wheels (output values are for wheel bottom points)/15(RT_tau_x) -> CoG rotation/21(RT_tau_x)
  Position and velocity of the wheels (output values are for wheel bottom points)/16(RT_tau_z) -> CoG rotation/22(RT_tau_z)
  [F_sigma_zr] -> CoG rotation/1(F_sigma_zr)
  [F_sigma_zf] -> CoG rotation/2(F_sigma_zf)
  [F_sigma_xr] -> CoG rotation/3(F_sigma_xr)
  [F_sigma_xf] -> CoG rotation/4(F_sigma_xf)
  [F_tau_zr] -> CoG rotation/11(F_tau_zr)
  [F_tau_zf] -> CoG rotation/12(F_tau_zf)
  [F_tau_xr] -> CoG rotation/13(F_tau_xr)
  [F_tau_xf] -> CoG rotation/14(F_tau_xf)
  F_sigma_anglef/1 -> Position and velocity of the wheels (output values are for wheel bottom points)/7(F_sigma_anglef)
  F_tau_anglef/1 -> Position and velocity of the wheels (output values are for wheel bottom points)/8(F_tau_anglef)
  F_sigma_angler/1 -> Position and velocity of the wheels (output values are for wheel bottom points)/9(F_sigma_angler)
  F_tau_angler/1 -> Position and velocity of the wheels (output values are for wheel bottom points)/10(F_tau_angler)
  [FT_z] -> Ground properties update for tines/8(FT_z)
  [F_tine_depth] -> Ground properties update for tines/11(F_tine_depth)
  sr_r/1 -> Ground properties update for tines/9(sr_r)
  [F_tine_x] -> Ground properties update for tines/10(F_tine_x)
  [FT_x] -> Ground properties update for tines/7(FT_x)
  Ground properties update for rear tire/3(index_upd_low) -> Ground properties update for tines/5(index_upd_low)
  Ground properties update for rear tire/2(index_upd_high) -> Ground properties update for tines/6(index_upd_high)
  [B_tine_x] -> Ground properties update for tines/12(B_tine_x)
  [B_tine_depth] -> Ground properties update for tines/13(B_tine_depth)
  Towed tool calculations/5(F_tine_depth) -> [F_tine_depth]
  Towed tool calculations/6(B_tine_depth) -> [B_tine_depth]
  Towed tool calculations/7(F_tine_x) -> [F_tine_x]
  Towed tool calculations/8(B_tine_x) -> [B_tine_x]
  Ground properties update for tines/1(F_tine_upd_params) -> Towed tool calculations/11(F_tine_upd_params)
  Ground properties update for tines/2(B_tine_upd_params) -> Towed tool calculations/10(B_tine_upd_params)
  Ground properties update for rear tire/7(upd_kx) -> Ground properties update for tines/1(upd_kx)
  Ground properties update for rear tire/6(upd_coh) -> Ground properties update for tines/2(upd_coh)
  Ground properties update for rear tire/5(upd_rho) -> Ground properties update for tines/3(upd_rho)
  Ground properties update for rear tire/4(upd_h) -> Ground properties update for tines/4(upd_h)
  Towed tool calculations/1(F_hook_x) -> Gain/1
  Towed tool calculations/2(F_hook_z) -> Gain1/1

== system eAgriBot_V4/Driver/Control ==
  sr_r : Inport
  sr_f : Inport  Port=2
  v_ref : Inport  Port=3
  v_error : Inport  Port=4
  Constant{,1..3} (4 alike) : Constant  Value=0
  Constant4 : Constant  Value=drivetype
  Constant5 : Constant  Value=sr_lim_slip_f
  Constant6 : Constant  Value=sr_lim_skid
  Constant7 : Constant  Value=sr_lim_slip_r
  Constant8 : Constant  Value=T_multi_r
  PID Controller : slpidlib/PID Controller  Controller=PID  Form=Parallel  TimeDomain=Continuous-time  UseExternalTs=off  SampleTime=-1  IntegratorMethod=Forward Euler  FilterMethod=Forward Euler  ControllerParametersSource=internal  P=P_gain  I=I_gain  UseKiTs=off  D=0  N=100  UseFilter=on  TunerSelectOption=Transfer Function Based (PID Tuner App)  InitialConditionSource=internal  InitialConditionForIntegrator=0  InitialConditionForFilter=0  DifferentiatorICPrevScaledInput=0  ExternalReset=none  TrackingMode=off  Kt=1  LimitOutput=on  SatLimitsSource=internal  UpperSaturationLimit=1  LowerSaturationLimit=-1  LinearizeAsGain=on  AntiWindupMode=none  Kb=1/P_gain  LimitIntegrator=off  UpperIntegratorSaturationLimit=inf  LowerIntegratorSaturationLimit=-inf  POutMin=[]  POutMax=[]  IOutMin=[]  IOutMax=[]  DOutMin=[]  DOutMax=[]  NOutMin=[]  NOutMax=[]  SumOutMin=[]  SumOutMax=[]  SaturationOutMin=[]  SaturationOutMax=[]  PParamMin=[]  PParamMax=[]  IParamMin=[]  IParamMax=[]  DParamMin=[]  DParamMax=[]  NParamMin=[]  NParamMax=[]  KbParamMin=[]  KbParamMax=[]  KtParamMin=[]  KtParamMax=[]  KbOutMin=[]  KbOutMax=[]  KtOutMin=[]  KtOutMax=[]  IntegratorOutMin=[]  IntegratorOutMax=[]  FilterOutMin=[]  FilterOutMax=[]  SumI1OutMin=[]  SumI1OutMax=[]  SumI2OutMin=[]  SumI2OutMax=[]  SumI3OutMin=[]  SumI3OutMax=[]  SumI4OutMin=[]  SumI4OutMax=[]  SumDOutMin=[]  SumDOutMax=[]  DifferentiatorOutMin=[]  DifferentiatorOutMax=[]  FilterDiffOutCoefMin=[]  FilterDiffOutCoefMax=[]  ReciprocalOutMin=[]  ReciprocalOutMax=[]  SumDenOutMin=[]  SumDenOutMax=[]  SumNumOutMin=[]  SumNumOutMax=[]  DivideOutMin=[]  DivideOutMax=[]  UdiffTsProdOutMin=[]  UdiffTsProdOutMax=[]  NTsProdOutMin=[]  NTsProdOutMax=[]  UintegralTsProdOutMin=[]  UintegralTsProdOutMax=[]  UngainTsProdOutMin=[]  UngainTsProdOutMax=[]  ClampingZeroOutDataTypeStr=Inherit: Inherit via back propagation  ClampingZeroOutMin=[]  ClampingZeroOutMax=[]  FilterDenConstantOutDataTypeStr=Inherit: Inherit via back propagation  FilterDenConstantOutMin=[]  FilterDenConstantOutMax=[]  PCopyOutDataTypeStr=Inherit: Inherit via back propagation  PCopyOutMin=[]  PCopyOutMax=[]  NCopyOutDataTypeStr=Inherit: Inherit via back propagation  NCopyOutMin=[]  NCopyOutMax=[]  IntegratorContinuousStateAttributes=''  IntegratorStateMustResolveToSignalObject=off  IntegratorRTWStateStorageClass=Auto  FilterContinuousStateAttributes=''  FilterStateMustResolveToSignalObject=off  FilterRTWStateStorageClass=Auto  ParallelPVariant=InternalParameters  IdealPVariant=Disabled  IVariant=InternalParameters  DVariant=InternalParameters  IntegratorVariant=Continuous  SatVariant=Enabled  AWVariant=Passthrough  PCopyVariant=Disabled  TRVariant=Disabled  FdbkBlocksVariant=Forward  IdealPFdbkVariant=Disabled  SatFdbkVariant=Disabled  DerivativeFilterVariant=ContFilter  NVariant=InternalParameters  NCopyVariant=Disabled  FilterICVariant=InternalICsFilter  IntegratorICVariant=InternalICs  ExternalResetVariant=Disabled  TRSumVariant=Passthrough  SumFdbkVariant=Disabled  SumVariant=Sum_PID  TsampFilterVariant=InternalTs  TsampNgainVariant=Passthrough  TsampIntegralVariant=Passthrough  ExternalSaturationOutDataTypeStr=Inherit: Same as second input
  Switch{,1,3..4} (4 alike) : Switch  SaturateOnIntegerOverflow=off  InputSameDT=off
  Switch2 : Switch  Criteria=u2 > Threshold  SaturateOnIntegerOverflow=off  InputSameDT=off
  Switch5 : Switch  Criteria=u2 > Threshold  SaturateOnIntegerOverflow=off  InputSameDT=off
  To Workspace1 : ToWorkspace  VariableName=throttle_f  SaveFormat=Timeseries  SampleTime=-1
  To Workspace2 : ToWorkspace  VariableName=throttle  SaveFormat=Timeseries  SampleTime=-1
  To Workspace3 : ToWorkspace  VariableName=brake_f  SaveFormat=Timeseries  SampleTime=-1
  To Workspace4 : ToWorkspace  VariableName=brake  SaveFormat=Timeseries  SampleTime=-1
  Torque limit based on slip : MATLAB Function  TreatAsAtomicUnit=on  SystemSampleTime=step_size
  throttle_r : Outport
  brake_r : Outport  Port=2
  throttle_f : Outport  Port=3
  brake_f : Outport  Port=4
  wires:
  Switch/1 -> Switch2/1
  sr_r/1 -> Torque limit based on slip/1(sr_r)
  Constant/1 -> Switch2/3, Switch/3
  v_error/1 -> PID Controller/1
  Switch1/1 -> brake_r/1, To Workspace4/1
  Constant1/1 -> Switch1/1
  Constant6/1 -> Torque limit based on slip/5(sr_lim_skid)
  Switch2/1 -> throttle_r/1, To Workspace2/1
  v_ref/1 -> Switch5/2, Switch2/2
  Constant5/1 -> Torque limit based on slip/3(sr_lim_slip_f)
  Torque limit based on slip/1(control_lim_r) -> Switch1/2, Switch1/3, Switch/1, Switch/2
  PID Controller/1 -> Torque limit based on slip/6(control)
  sr_f/1 -> Torque limit based on slip/2(sr_f)
  Torque limit based on slip/2(control_lim_f) -> Switch4/2, Switch4/3, Switch3/1, Switch3/2
  Switch4/1 -> brake_f/1, To Workspace3/1
  Constant3/1 -> Switch4/1
  Constant2/1 -> Switch5/3, Switch3/3
  Switch5/1 -> throttle_f/1, To Workspace1/1
  Switch3/1 -> Switch5/1
  Constant4/1 -> Torque limit based on slip/7(drivetype)
  Constant7/1 -> Torque limit based on slip/4(sr_lim_slip_r)
  Constant8/1 -> Torque limit based on slip/8(T_multi_r)

== system eAgriBot_V4/Driver/Main cycle ==
  end_time_precycle : Inport
  v_ms : Inport  Port=2
  Clock : Clock
  Clock2 : Clock
  Clock3 : Clock
  Constant11 : Constant  Value=main_cycle_delay
  Constant12 : Constant  Value=main_cycle_delay
  Constant3 : Constant  Value=decel_begin_dist
  Constant4 : Constant  Value=decel
  Constant5 : Constant  Value=vel_max/3.6
  Constant6 : Constant  Value=0
  Data Type Conversion1 : DataTypeConversion  OutDataTypeStr=double  SaturateOnIntegerOverflow=off  RndMeth=Floor
  Deceleration : MATLAB Function  TreatAsAtomicUnit=on  SystemSampleTime=step_size
  Delay : Delay  DelayLength=1  SampleTime=step_size
  Delay1 : Delay  DelayLength=1  SampleTime=step_size
  Delay6 : Delay  DelayLength=1  InitialCondition=0  SampleTime=step_size
  Delay7 : Delay  DelayLength=1  InitialCondition=9999  SampleTime=step_size
  Gain : Gain  Gain=accel
  Integrator : Integrator
  Relational Operator : RelationalOperator  Operator=<  OutDataTypeStr=boolean  RndMeth=Simplest  InputSameDT=off
  Saturation : Saturate  UpperLimit=vel_max/3.6  LowerLimit=0
  Sum1 : Sum  Inputs=|+-
  Sum2 : Sum  Inputs=|+-
  Sum3 : Sum  Inputs=|++
  Switch4 : Switch  Threshold=decel_begin_dist  SaturateOnIntegerOverflow=off  InputSameDT=off
  Switch5 : Switch  Criteria=u2 ~= 0  SaturateOnIntegerOverflow=off  InputSameDT=off
  To Workspace : ToWorkspace  VariableName=precycle_endtime  SampleTime=-1
      settings: MaxDataPoints=1
  To Workspace1 : ToWorkspace  VariableName=maincycle_dbegintime  SampleTime=-1
      settings: MaxDataPoints=1
  end_time_new : Outport
  v_ref_maincycle : Outport  Port=2
  main_cycle_on_check : Outport  Port=3
  wires:
  Switch4/1 -> v_ref_maincycle/1
  Integrator/1 -> Deceleration/5(cur_dist), Switch4/2
  Delay/1 -> Deceleration/6(check)
  Switch5/1 -> Integrator/1
  Constant12/1 -> Sum3/2
  Deceleration/4(end_time_new) -> end_time_new/1, Delay7/1
  Clock/1 -> Deceleration/1(clock)
  Data Type Conversion1/1 -> Switch5/2
  Delay1/1 -> Deceleration/7(time_d_begin)
  Constant4/1 -> Deceleration/3(d)
  Delay7/1 -> Deceleration/8(end_time)
  Saturation/1 -> Switch4/3
  Deceleration/1(v_target) -> Switch4/1
  end_time_precycle/1 -> To Workspace/1, Sum3/1, Relational Operator/1
  Constant5/1 -> Deceleration/4(v_max)
  Constant3/1 -> Deceleration/2(d_begin_dist)
  Sum1/1 -> Relational Operator/2
  Deceleration/2(check_new) -> Delay/1
  Deceleration/3(time_d_begin_new) -> Delay1/1, To Workspace1/1
  Sum2/1 -> main_cycle_on_check/1, Gain/1
  Clock2/1 -> Sum1/1
  Relational Operator/1 -> Data Type Conversion1/1
  Constant6/1 -> Switch5/3
  Constant11/1 -> Sum1/2
  v_ms/1 -> Switch5/1
  Sum3/1 -> Sum2/2
  Clock3/1 -> Sum2/1
  Gain/1 -> Saturation/1
  Deceleration/5(isover_new) -> Delay6/1
  Delay6/1 -> Deceleration/9(isover)

== system eAgriBot_V4/Driver/Pre-cycle ==
  v_ms : Inport
  Clock1 : Clock
  Constant10 : Constant  Value=pre_vel/3.6
  Constant8 : Constant  Value=pre_decel_begin_dist
  Constant9 : Constant  Value=pre_decel
  Deceleration1 : MATLAB Function  TreatAsAtomicUnit=on  SystemSampleTime=step_size
  Delay2 : Delay  DelayLength=1  SampleTime=step_size
  Delay3 : Delay  DelayLength=1  SampleTime=step_size
  Delay4 : Delay  DelayLength=1  InitialCondition=0  SampleTime=step_size
  Delay5 : Delay  DelayLength=1  InitialCondition=9999  SampleTime=step_size
  Integrator1 : Integrator
  Ramp1 : simulink/Sources/Ramp  slope=pre_accel  start=pre_start  InitialOutput=0
  Saturation1 : Saturate  UpperLimit=5/3.6  LowerLimit=0
  Switch3 : Switch  Threshold=pre_decel_begin_dist  SaturateOnIntegerOverflow=off  InputSameDT=off
  end_time_new : Outport
  v_ref_precycle : Outport  Port=2
  wires:
  Deceleration1/2(check_new) -> Delay2/1
  Integrator1/1 -> Deceleration1/5(cur_dist), Switch3/2
  Delay2/1 -> Deceleration1/6(check)
  Constant9/1 -> Deceleration1/3(d)
  Delay3/1 -> Deceleration1/7(time_d_begin)
  Clock1/1 -> Deceleration1/1(clock)
  Ramp1/1 -> Saturation1/1
  Deceleration1/3(time_d_begin_new) -> Delay3/1
  Constant8/1 -> Deceleration1/2(d_begin_dist)
  Delay5/1 -> Deceleration1/8(end_time)
  Constant10/1 -> Deceleration1/4(v_max)
  Saturation1/1 -> Switch3/3
  Deceleration1/1(v_target) -> Switch3/1
  Delay4/1 -> Deceleration1/9(isover)
  Deceleration1/5(isover_new) -> Delay4/1
  v_ms/1 -> Integrator1/1
  Switch3/1 -> v_ref_precycle/1
  Deceleration1/4(end_time_new) -> end_time_new/1, Delay5/1

== system eAgriBot_V4/Driver/Stop simulation ==
  main_cycle_endtime : Inport
  Clock4 : Clock
  Clock5 : Clock
  Constant13 : Constant  Value=0
  Constant2 : Constant  Value=end_delay
  Constant7 : Constant
  Stop Simulation : Stop
  Sum4 : Sum  Inputs=|+-
  Sum5 : Sum  Inputs=|+-
  Switch7 : Switch  SaturateOnIntegerOverflow=off  InputSameDT=off
  Switch8 : Switch  Threshold=simu_max_time  SaturateOnIntegerOverflow=off  InputSameDT=off
  wires:
  Constant7/1 -> Switch7/1, Switch8/1
  Clock4/1 -> Sum4/1
  Constant2/1 -> Sum4/2
  Clock5/1 -> Switch8/2
  Switch7/1 -> Switch8/3
  Sum4/1 -> Sum5/1
  Constant13/1 -> Switch7/3
  Sum5/1 -> Switch7/2
  Switch8/1 -> Stop Simulation/1
  main_cycle_endtime/1 -> Sum5/2

== system eAgriBot_V4/Vehicle dynamics/CoG X dynamics ==
  F_sigma_xf : Inport
  F_tau_xf : Inport  Port=2
  F_sigma_xr : Inport  Port=3
  F_tau_xr : Inport  Port=4
  F_hook_x : Inport  Port=5
  CoG s_x : Integrator  InitialCondition=s_init
  CoG v_x : Integrator  InitialCondition=v_init  LowerSaturationLimit=0
  Gain : Gain  Gain=1/m
  Sum : Sum  Inputs=+++++
  To Workspace : ToWorkspace  VariableName=v_ms  SaveFormat=Timeseries  SampleTime=-1
  To Workspace1 : ToWorkspace  VariableName=a_x  SaveFormat=Timeseries  SampleTime=-1
  CoG_a_x : Outport
  CoG_v_x : Outport  Port=2
  CoG_s_x : Outport  Port=3
  wires:
  Gain/1 -> To Workspace1/1, CoG_a_x/1, CoG v_x/1
  CoG v_x/1 -> To Workspace/1, CoG_v_x/1, CoG s_x/1
  CoG s_x/1 -> CoG_s_x/1
  F_sigma_xf/1 -> Sum/1
  F_tau_xf/1 -> Sum/2
  F_hook_x/1 -> Sum/5
  F_tau_xr/1 -> Sum/4
  F_sigma_xr/1 -> Sum/3
  Sum/1 -> Gain/1

== system eAgriBot_V4/Vehicle dynamics/CoG Z dynamics ==
  F_sigma_zf : Inport
  F_tau_zf : Inport  Port=2
  F_hook_z : Inport  Port=3
  F_sigma_zr : Inport  Port=4
  F_tau_zr : Inport  Port=5
  CoG s_z : Integrator  InitialCondition=init_CoG_height
  CoG v_z : Integrator  InitialCondition=init_CoG_v_z
  Constant : Constant  Value=m*g
  Gain1 : Gain  Gain=1/m
  Sum : Sum  Inputs=+++++
  Sum2 : Sum  Inputs=|+-
  CoG_a_z : Outport
  CoG_v_z : Outport  Port=2
  CoG_s_z : Outport  Port=3
  wires:
  Gain1/1 -> CoG_a_z/1, CoG v_z/1
  Constant/1 -> Sum2/2
  CoG v_z/1 -> CoG_v_z/1, CoG s_z/1
  CoG s_z/1 -> CoG_s_z/1
  Sum/1 -> Sum2/1
  F_sigma_zf/1 -> Sum/1
  F_tau_zf/1 -> Sum/2
  F_sigma_zr/1 -> Sum/3
  F_tau_zr/1 -> Sum/4
  Sum2/1 -> Gain1/1
  F_hook_z/1 -> Sum/5
